simulink model "Sim_1_MPC_Robot_PS_sing_shooting_siml"  (R2022b)
settings: Solver=VariableStepAuto  StartTime=0.0  StopTime=6  RelTol=1e-3
libraries: robotmobilelib x1, mobileRoboticsLib x1
settings Model: Creator=quran  LastModifiedBy=quran

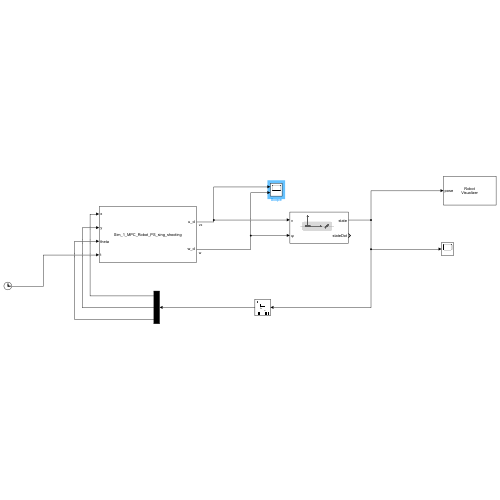
[thumbnail: Simulink's stored preview of the top-level diagram]
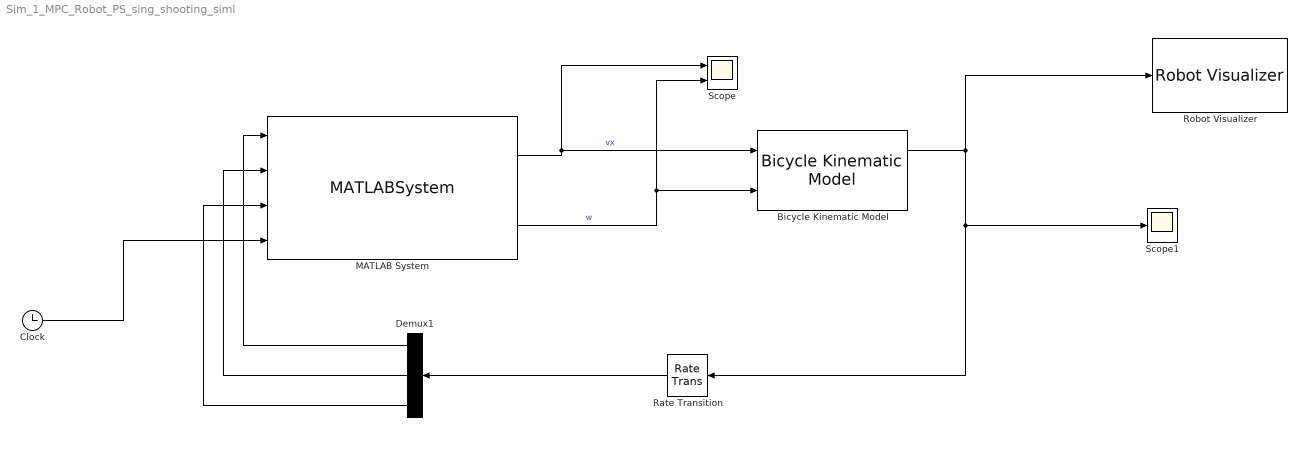
== system Sim_1_MPC_Robot_PS_sing_shooting_siml ==
  Bicycle Kinematic Model : robotmobilelib/Bicycle Kinematic Model  VehicleInputs=Vehicle Speed & Steering Angle  WheelBase=1  VehicleSpeedRange=[-inf inf]  MaxSteeringAngle=pi/4  InitialState=[0; 0; 0]  SimulateUsing=Interpreted execution
  Clock : Clock
  Demux1 : Demux  Outputs=3
  MATLAB System : MATLABSystem  System=Sim_1_MPC_Robot_PS_sing_shooting  SimulateUsing=Interpreted execution
      mask Type: Sim_1_MPC_Robot_PS_sing_shooting
      mask Display:
      | disp('Sim_1_MPC_Robot_PS_sing_shooting');
      | port_label('input',1,'x');
      | port_label('input',2,'y');
      | port_label('input',3,'theta');
      | port_label('input',4,'t');
      | port_label('output',1,'u_cl');
      | port_label('output',2,'w_cl');
  Rate Transition : RateTransition
  Robot Visualizer : mobileRoboticsLib/Environments/Robot Visualizer  robotRadius=0  showTrajectory=on  hasWaypoints=off  hasLidar=off  sensorOffset=[ 0, 0 ]  scanAngles=[ -pi/4, 0, pi/4 ]  hasObjDetector=off  objDetectorOffset=[ 0, 0 ]  objDetectorAngle=0  objDetectorFOV=pi/4  objDetectorMaxRange=5  objectColors=[ 1, 0, 0; 0, 1, 0; 0, 0, 1 ]  objectMarkers=s
  Scope : Scope  NumInputPorts=2
  Scope1 : Scope
  wires:
  MATLAB System/2 -> Bicycle Kinematic Model/2, Scope/2  "w"
  Demux1/1 -> MATLAB System/1
  Demux1/2 -> MATLAB System/2
  Demux1/3 -> MATLAB System/3
  Rate Transition/1 -> Demux1/1
  MATLAB System/1 -> Scope/1, Bicycle Kinematic Model/1  "vx"
  Bicycle Kinematic Model/1 -> Robot Visualizer/1, Rate Transition/1, Scope1/1
  Clock/1 -> MATLAB System/4
